simulink model "Rebuild"  (R2024b)
settings: Solver=VariableStepAuto  StartTime=0.0  StopTime=12  RelTol=1e-3
values from neighbouring files (symbols this model uses):
  A = 1.1    [RT14e_Parameters.m]    (also in RT15e_Parameters.m = 1.088; RT15evo_Parameters.m = 1.088)
  Aero_balance = 55    [RT14e_Parameters.m]    (also in RT15e_Parameters.m; RT15evo_Parameters.m)
  Aeromaps_ON = 0    [SIM_setup.m]
  air_density = 1.2    [SIM_setup.m]
  Balance_FW = Data_FW_STD(1:end,2)    [RT15e_Parameters.m]    (also in RT15evo_Parameters.m)
  Balance_R_11 = Data_R_11(1:end,2)    [RT15e_Parameters.m]    (also in RT15evo_Parameters.m)
  Br_coef_of_friction_F = 0.33    [RT14e_Parameters.m]    (also in RT15e_Parameters.m; RT15evo_Parameters.m)
  Br_coef_of_friction_R = 0.33    [RT14e_Parameters.m]    (also in RT15e_Parameters.m; RT15evo_Parameters.m)
  Br_pistons_area_F = 3617.26/1e6    (= 0.00361726)    [RT14e_Parameters.m]    (also in RT15e_Parameters.m; RT15evo_Parameters.m)
  Br_pistons_area_R = 2026.83/1e6    (= 0.00202683)    [RT14e_Parameters.m]    (also in RT15e_Parameters.m; RT15evo_Parameters.m)
  CdA = 1.31*A    (= 1.441)    [RT14e_Parameters.m]    (also in RT15e_Parameters.m = 1.700544; RT15evo_Parameters.m = 1.700544)
  CdA_FW = Data_FW_STD(1:end,3)    [RT15e_Parameters.m]    (also in RT15evo_Parameters.m)
  CdA_R_11 = Data_R_11(1:end,3)    [RT15e_Parameters.m]    (also in RT15evo_Parameters.m)
  ClA = 3.3*A    (= 3.63)    [RT14e_Parameters.m]    (also in RT15e_Parameters.m = 4.36288; RT15evo_Parameters.m = 4.36288)
  ClA_FW = Data_FW_STD(1:end,4)    [RT15e_Parameters.m]    (also in RT15evo_Parameters.m)
  ClA_R_11 = Data_R_11(1:end,4)    [RT15e_Parameters.m]    (also in RT15evo_Parameters.m)
  CoG_z = 0.35    [RT14e_Parameters.m]    (also in RT15e_Parameters.m = 0.28495; RT15evo_Parameters.m = 0.28495)
  Default_Fz_FL = Default_Fz_F/2 + (Default_Fz_F*CoG_y/Track_Front)    [RT14e_Parameters.m]    (also in RT15e_Parameters.m; RT15evo_Parameters.m)
  Default_Fz_FR = Default_Fz_F/2 - (Default_Fz_F*CoG_y/Track_Front)    [RT14e_Parameters.m]    (also in RT15e_Parameters.m; RT15evo_Parameters.m)
  Default_Fz_RL = Default_Fz_R/2 + (Default_Fz_R*CoG_y/Track_Rear)    [RT14e_Parameters.m]    (also in RT15e_Parameters.m; RT15evo_Parameters.m)
  Default_Fz_RR = Default_Fz_R/2 - (Default_Fz_R*CoG_y/Track_Rear)    [RT14e_Parameters.m]    (also in RT15e_Parameters.m; RT15evo_Parameters.m)
  Effective_br_disk_r_F = 0.0905    [RT14e_Parameters.m]    (also in RT15e_Parameters.m; RT15evo_Parameters.m)
  Effective_br_disk_r_R = 0.0895    [RT14e_Parameters.m]    (also in RT15e_Parameters.m; RT15evo_Parameters.m)
  Front_brake_balance = 0.0    (= 0)    [RT14e_Parameters.m]    (also in RT15e_Parameters.m; RT15evo_Parameters.m)
  Front_brake_pump_area = 153.94    [RT14e_Parameters.m]    (also in RT15e_Parameters.m; RT15evo_Parameters.m)
  Front_desired_brake_p_balance = 0.6    [RT14e_Parameters.m]    (also in RT15e_Parameters.m; RT15evo_Parameters.m)
  FW_Setup = Data_FW_STD(1:end,1)    [RT15e_Parameters.m]    (also in RT15evo_Parameters.m)
  Fx = Data_Fx(2:end,3:end)    [RT14e_Parameters.m]    (also in RT15e_Parameters.m; RT15evo_Parameters.m)
  Fy = Data_Fy(2:end,3:end)    [RT14e_Parameters.m]    (also in RT15e_Parameters.m; RT15evo_Parameters.m)
  Fz = Data_Fy(2:end,2)    [RT14e_Parameters.m]    (also in RT15e_Parameters.m; RT15evo_Parameters.m)
  g = 9.81    [SIM_setup.m]
  Gear_ratio = 12.9    [RT14e_Parameters.m]    (also in RT15e_Parameters.m; RT15evo_Parameters.m)
  Iz_wehicle = 120    [RT14e_Parameters.m]    (also in RT15e_Parameters.m; RT15evo_Parameters.m)
  Iz_wheel = 0.15    [RT14e_Parameters.m]    (also in RT15e_Parameters.m; RT15evo_Parameters.m)
  Lf = Wheelbase - CoG_x    (= 0.77)    [RT14e_Parameters.m]    (also in RT15e_Parameters.m = 0.7504; RT15evo_Parameters.m = 0.7504)
  LLTD = 0.45    [RT14e_Parameters.m]    (also in RT15e_Parameters.m = 0.55; RT15evo_Parameters.m = 0.55)
  Lock_brake_balance = false    [RT14e_Parameters.m]    (also in RT15e_Parameters.m; RT15evo_Parameters.m)
  Lr = Wheelbase - Lf    (= 0.755)    [RT14e_Parameters.m]    (also in RT15e_Parameters.m = 0.7746; RT15evo_Parameters.m = 0.7746)
  Mass = Vehicle_mass + Driver_mass    (= 290)    [RT14e_Parameters.m]    (also in RT15e_Parameters.m = 265; RT15evo_Parameters.m)
  Motor_maximum_power = 35366    [RT14e_Parameters.m]    (also in RT15e_Parameters.m; RT15evo_Parameters.m)
  RB_torque_setting_1 = -2    [RT14e_Parameters.m]    (also in RT15e_Parameters.m; RT15evo_Parameters.m)
  RB_torque_setting_10 = -20    [RT14e_Parameters.m]    (also in RT15e_Parameters.m; RT15evo_Parameters.m)
  RB_torque_setting_2 = -4    [RT14e_Parameters.m]    (also in RT15e_Parameters.m; RT15evo_Parameters.m)
  RB_torque_setting_3 = -6    [RT14e_Parameters.m]    (also in RT15e_Parameters.m; RT15evo_Parameters.m)
  RB_torque_setting_4 = -8    [RT14e_Parameters.m]    (also in RT15e_Parameters.m; RT15evo_Parameters.m)
  RB_torque_setting_5 = -10    [RT14e_Parameters.m]    (also in RT15e_Parameters.m; RT15evo_Parameters.m)
  RB_torque_setting_6 = -12    [RT14e_Parameters.m]    (also in RT15e_Parameters.m; RT15evo_Parameters.m)
  RB_torque_setting_7 = -14    [RT14e_Parameters.m]    (also in RT15e_Parameters.m; RT15evo_Parameters.m)
  RB_torque_setting_8 = -16    [RT14e_Parameters.m]    (also in RT15e_Parameters.m; RT15evo_Parameters.m)
  RB_torque_setting_9 = -18    [RT14e_Parameters.m]    (also in RT15e_Parameters.m; RT15evo_Parameters.m)
  Rear_brake_pump_area = 198.56    [RT14e_Parameters.m]    (also in RT15e_Parameters.m; RT15evo_Parameters.m)
  Roll_Angle_11 = Data_R_11(1:end,1)    [RT15e_Parameters.m]    (also in RT15evo_Parameters.m)
  SA = Data_Fy(1,3:end)    [RT14e_Parameters.m]    (also in RT15e_Parameters.m; RT15evo_Parameters.m)
  SR = Data_Fx(1,3:end)    [RT14e_Parameters.m]    (also in RT15e_Parameters.m; RT15evo_Parameters.m)
  start_acc_x = double(start_acc_x_ts.Data)    [SIM_setup.m]
  start_acc_y = double(start_acc_y_ts.Data)    [SIM_setup.m]
  start_time = 1188    [SIM_setup.m]
  start_velocity_x = double(start_velocity_x_ts.Data)    [SIM_setup.m]
  start_velocity_y = double(start_velocity_y_ts.Data)    [SIM_setup.m]
  start_yaw_acc = double(start_yaw_acc_ts.Data)    [SIM_setup.m]
  start_yaw_rate = double(start_yaw_rate_ts.Data)    [SIM_setup.m]
  Static_Camber_FL = 0    [RT14e_Parameters.m]    (also in RT15e_Parameters.m; RT15evo_Parameters.m)
  Static_Camber_FR = 0    [RT14e_Parameters.m]    (also in RT15e_Parameters.m; RT15evo_Parameters.m)
  Static_Camber_RL = 0    [RT14e_Parameters.m]    (also in RT15e_Parameters.m; RT15evo_Parameters.m)
  Static_Camber_RR = 0    [RT14e_Parameters.m]    (also in RT15e_Parameters.m; RT15evo_Parameters.m)
  Static_Toe_FL = 0    [RT14e_Parameters.m]    (also in RT15e_Parameters.m; RT15evo_Parameters.m)
  Static_Toe_FR = 0    [RT14e_Parameters.m]    (also in RT15e_Parameters.m; RT15evo_Parameters.m)
  Static_Toe_RL = 0    [RT14e_Parameters.m]    (also in RT15e_Parameters.m; RT15evo_Parameters.m)
  Static_Toe_RR = 0    [RT14e_Parameters.m]    (also in RT15e_Parameters.m; RT15evo_Parameters.m)
  Steering_Angle_FL = Data_Steering(1:end,2)    [RT14e_Parameters.m]    (also in RT15e_Parameters.m; RT15evo_Parameters.m)
  Steering_Angle_FR = Data_Steering(1:end,3)    [RT14e_Parameters.m]    (also in RT15e_Parameters.m; RT15evo_Parameters.m)
  Steering_Wheel_Angle = Data_Steering(1:end,1)    [RT14e_Parameters.m]    (also in RT15e_Parameters.m; RT15evo_Parameters.m)
  Tire_radius = 0.203    [RT14e_Parameters.m]    (also in RT15e_Parameters.m; RT15evo_Parameters.m)
  Torque_limit_2 = Motor_maximum_torque*0.2    (= 5.82)    [RT14e_Parameters.m]    (also in RT15e_Parameters.m; RT15evo_Parameters.m)
  Torque_limit_3 = Motor_maximum_torque*0.3    (= 8.73)    [RT14e_Parameters.m]    (also in RT15e_Parameters.m; RT15evo_Parameters.m)
  Torque_limit_4 = Motor_maximum_torque*0.4    (= 11.64)    [RT14e_Parameters.m]    (also in RT15e_Parameters.m; RT15evo_Parameters.m)
  Torque_limit_5 = Motor_maximum_torque*0.5    (= 14.55)    [RT14e_Parameters.m]    (also in RT15e_Parameters.m; RT15evo_Parameters.m)
  Torque_limit_6 = Motor_maximum_torque*0.6    (= 17.46)    [RT14e_Parameters.m]    (also in RT15e_Parameters.m; RT15evo_Parameters.m)
  Torque_limit_7 = Motor_maximum_torque*0.7    (= 20.37)    [RT14e_Parameters.m]    (also in RT15e_Parameters.m; RT15evo_Parameters.m)
  Torque_limit_8 = Motor_maximum_torque*0.8    (= 23.28)    [RT14e_Parameters.m]    (also in RT15e_Parameters.m; RT15evo_Parameters.m)
  Torque_limit_9 = 29.1    [RT14e_Parameters.m]    (also in RT15e_Parameters.m; RT15evo_Parameters.m)
  Torque_limit_max = Motor_maximum_torque    (= 29.1)    [RT14e_Parameters.m]    (also in RT15e_Parameters.m; RT15evo_Parameters.m)
  Torque_limit_min = Motor_maximum_torque*0.1    (= 2.91)    [RT14e_Parameters.m]    (also in RT15e_Parameters.m; RT15evo_Parameters.m)
  Torque_limit_set = 10    [RT14e_Parameters.m]    (also in RT15e_Parameters.m; RT15evo_Parameters.m)
  Track_Front = 1.2    [RT14e_Parameters.m]    (also in RT15e_Parameters.m; RT15evo_Parameters.m)
  Track_Rear = 1.18    [RT14e_Parameters.m]    (also in RT15e_Parameters.m; RT15evo_Parameters.m)
  TV_ON = 0    [SIM_setup.m]
  TV_RB_understeer_gradient_1 = -0.5    [RT14e_Parameters.m]    (also in RT15e_Parameters.m; RT15evo_Parameters.m)
  TV_RB_understeer_gradient_10 = 0.005    [RT14e_Parameters.m]    (also in RT15e_Parameters.m; RT15evo_Parameters.m)
  TV_RB_understeer_gradient_2 = -0.1    [RT14e_Parameters.m]    (also in RT15e_Parameters.m; RT15evo_Parameters.m)
  TV_RB_understeer_gradient_3 = 0.08    [RT14e_Parameters.m]    (also in RT15e_Parameters.m; RT15evo_Parameters.m)
  TV_RB_understeer_gradient_4 = 0.06    [RT14e_Parameters.m]    (also in RT15e_Parameters.m; RT15evo_Parameters.m)
  TV_RB_understeer_gradient_5 = 0.05    [RT14e_Parameters.m]    (also in RT15e_Parameters.m; RT15evo_Parameters.m)
  TV_RB_understeer_gradient_6 = 0.04    [RT14e_Parameters.m]    (also in RT15e_Parameters.m; RT15evo_Parameters.m)
  TV_RB_understeer_gradient_7 = 0.03    [RT14e_Parameters.m]    (also in RT15e_Parameters.m; RT15evo_Parameters.m)
  TV_RB_understeer_gradient_8 = 0.02    [RT14e_Parameters.m]    (also in RT15e_Parameters.m; RT15evo_Parameters.m)
  TV_RB_understeer_gradient_9 = 0.01    [RT14e_Parameters.m]    (also in RT15e_Parameters.m; RT15evo_Parameters.m)
  TV_understeer_gradient_1 = -0.5    [RT14e_Parameters.m]    (also in RT15e_Parameters.m; RT15evo_Parameters.m)
  TV_understeer_gradient_10 = 0.002    [RT14e_Parameters.m]    (also in RT15e_Parameters.m; RT15evo_Parameters.m)
  TV_understeer_gradient_2 = -0.1    [RT14e_Parameters.m]    (also in RT15e_Parameters.m; RT15evo_Parameters.m)
  TV_understeer_gradient_3 = 0.06    [RT14e_Parameters.m]    (also in RT15e_Parameters.m; RT15evo_Parameters.m)
  TV_understeer_gradient_4 = 0.05    [RT14e_Parameters.m]    (also in RT15e_Parameters.m; RT15evo_Parameters.m)
  TV_understeer_gradient_5 = 0.04    [RT14e_Parameters.m]    (also in RT15e_Parameters.m; RT15evo_Parameters.m)
  TV_understeer_gradient_6 = 0.03    [RT14e_Parameters.m]    (also in RT15e_Parameters.m; RT15evo_Parameters.m)
  TV_understeer_gradient_7 = 0.02    [RT14e_Parameters.m]    (also in RT15e_Parameters.m; RT15evo_Parameters.m)
  TV_understeer_gradient_8 = 0.01    [RT14e_Parameters.m]    (also in RT15e_Parameters.m; RT15evo_Parameters.m)
  TV_understeer_gradient_9 = 0.005    [RT14e_Parameters.m]    (also in RT15e_Parameters.m; RT15evo_Parameters.m)
  Vx_APPS_ON = 1    [SIM_setup.m]
  Wheel_rolling_resistance = 0.055    [RT14e_Parameters.m]    (also in RT15e_Parameters.m; RT15evo_Parameters.m)
  Wheelbase = 1.525    [RT14e_Parameters.m]    (also in RT15e_Parameters.m; RT15evo_Parameters.m)
undefined symbols (not defined in the file or in its folder): Actual_Torque_Value_RL, Actual_Torque_Value_RR, aero_balance, APPS, Brake_Pressure_Front, Brake_Pressure_Rear, Cl, lateral_load_transfer_distribution, maths_GPS_Velocity, Max_Torque, rad, s, Steering_position, tire_radius, wheel_base, Wheel_Speed_RL, Wheel_Speed_RR, Xsens_MTI_670_accX, Xsens_MTI_670_accY, Xsens_MTI_670_gyrZ
libraries: simulink x30, simulink_extras x11, slpidlib x9, dspstat3 x4, slrealtimeloglib x1, aerolibconvert2 x1
(part 3 of 6)

== system Rebuild/Main/Wheels & Tires/Wheel Speeds/Wheel Speed RL ==
  Rolling Resistance : Inport
  Fx [N] : Inport  Port=2
  Torque [Nm] : Inport  Port=3
  Add1 : Sum  Inputs=--+-
  Bus Selector : BusSelector  OutputSignals=Brake Torque [Nm].Brake Torque RL [Nm],Motor Torque [Nm].Motor Torque RL [Nm]
  Bus Selector1 : BusSelector  OutputSignals=Rolling Resistance RL
  Bus Selector2 : BusSelector  OutputSignals=Fx RL [N]
  Constant4 : Constant  Value=Tire_radius
  Gain : Gain  Gain=Gear_ratio
  Gain1 : Gain  Gain=1/Iz_wheel
  Integrator2 : Integrator  InitialCondition=start_velocity_x / Tire_radius
  Product : Product
  Saturation : Saturate  UpperLimit=200  LowerLimit=-20
  Wheel Speed RL [rad/s] : Outport
  wires:
  Fx [N]/1 -> Bus Selector2/1
  Bus Selector2/1 -> Product/2  "<Fx RL [N]>"
  Rolling Resistance/1 -> Bus Selector1/1
  Saturation/1 -> Wheel Speed RL [rad/s]/1
  Torque [Nm]/1 -> Bus Selector/1
  Bus Selector1/1 -> Add1/4  "<Rolling Resistance RL>"
  Bus Selector/1 -> Add1/2  "<Brake Torque RL [Nm]>"
  Gain1/1 -> Integrator2/1
  Integrator2/1 -> Saturation/1
  Product/1 -> Add1/1
  Add1/1 -> Gain1/1
  Constant4/1 -> Product/1
  Bus Selector/2 -> Gain/1  "<Motor Torque RL [Nm]>"
  Gain/1 -> Add1/3

== system Rebuild/Main/Wheels & Tires/Wheel Speeds/Wheel Speed RR ==
  Rolling Resistance : Inport
  Fx [N] : Inport  Port=2
  Torque [Nm] : Inport  Port=3
  Add1 : Sum  Inputs=--+-
  Bus Selector : BusSelector  OutputSignals=Brake Torque [Nm].Brake Torque RR [Nm],Motor Torque [Nm].Motor Torque RR [Nm]
  Bus Selector1 : BusSelector  OutputSignals=Rolling Resistance RR
  Bus Selector2 : BusSelector  OutputSignals=Fx RR [N]
  Constant4 : Constant  Value=Tire_radius
  Gain : Gain  Gain=Gear_ratio
  Gain1 : Gain  Gain=1/Iz_wheel
  Integrator2 : Integrator  InitialCondition=start_velocity_x / Tire_radius
  Product : Product
  Saturation : Saturate  UpperLimit=200  LowerLimit=-20
  Wheel Speed RL [rad/s] : Outport
  wires:
  Bus Selector/2 -> Gain/1  "<Motor Torque RR [Nm]>"
  Add1/1 -> Gain1/1
  Integrator2/1 -> Saturation/1
  Gain1/1 -> Integrator2/1
  Bus Selector2/1 -> Product/2  "<Fx RR [N]>"
  Fx [N]/1 -> Bus Selector2/1
  Bus Selector/1 -> Add1/2  "<Brake Torque RR [Nm]>"
  Bus Selector1/1 -> Add1/4  "<Rolling Resistance RR>"
  Constant4/1 -> Product/1
  Product/1 -> Add1/1
  Torque [Nm]/1 -> Bus Selector/1
  Rolling Resistance/1 -> Bus Selector1/1
  Saturation/1 -> Wheel Speed RL [rad/s]/1
  Gain/1 -> Add1/3

== system Rebuild/Main/Powertrain/Motors/Control Algorithms/ABS ==
  Brake_Torque [Nm] : Inport
  Slip_Ratio : Inport  Port=2
  ABS_FL : Subsystem
  ABS_FR : Subsystem
  ABS_RL : Subsystem
  ABS_RR : Subsystem
  Bus Creator : BusCreator  Inputs=4
  Bus Selector : BusSelector  OutputSignals=Front.FL,Front.FR,Rear.RL,Rear.RR
  Bus Selector1 : BusSelector  OutputSignals=Slip_Ratio_FL,Slip_Ratio_FR,Slip_Ratio_RL,Slip_Ratio_RR
  ABS_Torque : Outport
  wires:
  Brake_Torque [Nm]/1 -> Bus Selector/1
  Slip_Ratio/1 -> Bus Selector1/1
  Bus Selector/1 -> ABS_FL/1(Torque IN)  "<FL>"
  Bus Selector1/1 -> ABS_FL/2(Slip_Ratio)  "<Slip_Ratio_FL>"
  Bus Selector/2 -> ABS_FR/1(Torque IN)  "<FR>"
  Bus Selector1/2 -> ABS_FR/2(Slip_Ratio)  "<Slip_Ratio_FR>"
  Bus Selector/3 -> ABS_RL/1(Torque IN)  "<RL>"
  Bus Selector1/3 -> ABS_RL/2(Slip_Ratio)  "<Slip_Ratio_RL>"
  Bus Selector/4 -> ABS_RR/1(Torque IN)  "<RR>"
  Bus Selector1/4 -> ABS_RR/2(Slip_Ratio)  "<Slip_Ratio_RR>"
  ABS_FL/1(ABS Torque OUT) -> Bus Creator/1  "FL"
  ABS_FR/1(ABS Torque OUT) -> Bus Creator/2  "FR"
  ABS_RL/1(ABS Torque OUT) -> Bus Creator/3  "RL"
  ABS_RR/1(ABS Torque OUT) -> Bus Creator/4  "RR"
  Bus Creator/1 -> ABS_Torque/1  "ABS_Torque"

== system Rebuild/Main/Powertrain/Motors/Control Algorithms/ABS1 ==
  Brake_Torque [Nm] : Inport
  Slip_Ratio : Inport  Port=2
  ABS_FL1 : Subsystem
  ABS_FR1 : Subsystem
  ABS_RL1 : Subsystem
  ABS_RR1 : Subsystem
  Bus Creator2 : BusCreator  Inputs=4
  Bus Selector2 : BusSelector  OutputSignals=Front.FL,Front.FR,Rear.RL,Rear.RR
  Bus Selector3 : BusSelector  OutputSignals=Slip_Ratio_FL,Slip_Ratio_FR,Slip_Ratio_RL,Slip_Ratio_RR
  ABS_Torque : Outport
  wires:
  Bus Creator2/1 -> ABS_Torque/1  "ABS_Torque"
  Bus Selector3/3 -> ABS_RL1/2(Slip_Ratio)  "<Slip_Ratio_RL>"
  Bus Selector3/2 -> ABS_FR1/2(Slip_Ratio)  "<Slip_Ratio_FR>"
  ABS_RR1/1(ABS Torque OUT) -> Bus Creator2/4  "RR"
  Bus Selector2/3 -> ABS_RL1/1(Torque IN)  "<RL>"
  Bus Selector2/2 -> ABS_FR1/1(Torque IN)  "<FR>"
  Bus Selector2/4 -> ABS_RR1/1(Torque IN)  "<RR>"
  ABS_FL1/1(ABS Torque OUT) -> Bus Creator2/1  "FL"
  ABS_FR1/1(ABS Torque OUT) -> Bus Creator2/2  "FR"
  Bus Selector3/4 -> ABS_RR1/2(Slip_Ratio)  "<Slip_Ratio_RR>"
  ABS_RL1/1(ABS Torque OUT) -> Bus Creator2/3  "RL"
  Bus Selector3/1 -> ABS_FL1/2(Slip_Ratio)  "<Slip_Ratio_FL>"
  Bus Selector2/1 -> ABS_FL1/1(Torque IN)  "<FL>"
  Brake_Torque [Nm]/1 -> Bus Selector2/1
  Slip_Ratio/1 -> Bus Selector3/1

== system Rebuild/Main/Powertrain/Motors/Control Algorithms/TV Algorithm ==
  Brakes : Inport
  Positive Torque Command [Nm] : Inport  Port=2
  States : Inport  Port=3
  Wheel Angle F [deg] : Inport  Port=4
  Bus Selector : BusSelector  OutputSignals=Yaw_Rate [rad/s],Y,X,V_x [m/s],V_y [m/s]
  Radians to Degrees : simulink_extras/Transformations/Radians to Degrees
  Subsystem : Subsystem
  Torque Vectoring : Subsystem
  Commanded Torque RL [Nm] : Outport
  Commanded Torque RR [Nm] : Outport  Port=2
  wires:
  States/1 -> Bus Selector/1
  Bus Selector/1 -> Radians to Degrees/1  "<Yaw_Rate [rad/s]>"
  Torque Vectoring/1(Torque After TV RL [Nm]) -> Commanded Torque RL [Nm]/1  "Torque After TV RL [Nm]"
  Torque Vectoring/2(Torque After TV RR [Nm]) -> Commanded Torque RR [Nm]/1  "Torque After TV RL [Nm]"
  Wheel Angle F [deg]/1 -> Torque Vectoring/8(Wheel Angle F [deg])
  Bus Selector/2 -> Torque Vectoring/5(Xsens accY [m/s2])  "<Y>"
  Bus Selector/3 -> Torque Vectoring/6(Xsens accX [m/s2])  "<X>"
  Bus Selector/4 -> Torque Vectoring/9(Vehicle Speed [km/h])  "<V_x [m/s]>"
  Positive Torque Command [Nm]/1 -> Torque Vectoring/2(Positive Torque Command RR [Nm]), Torque Vectoring/1(Positive Torque Command RL [Nm])
  Brakes/1 -> Torque Vectoring/7(Brakes)

== system Rebuild/Main/Powertrain/Motors/Power Limit/Power Calculation ==
  In1 : Inport
  Bus Creator : BusCreator  Inputs=4
  Bus Selector : BusSelector  OutputSignals=Motor Torque FL after TV [Nm]
  Bus Selector1 : BusSelector  OutputSignals=Motor Torque FR after TV [Nm]
  Bus Selector2 : BusSelector  OutputSignals=Wheel Speeds.Wheel Speeds [rad/s].Wheel Speed FL [rad/s]
  Bus Selector3 : BusSelector  OutputSignals=Wheel Speeds.Wheel Speeds [rad/s].Wheel Speed FR [rad/s]
  Bus Selector4 : BusSelector  OutputSignals=Motor Torque RL after TV [Nm]
  Bus Selector5 : BusSelector  OutputSignals=Wheel Speeds.Wheel Speeds [rad/s].Wheel Speed RL [rad/s]
  Bus Selector6 : BusSelector  OutputSignals=Motor Torque RR after TV [Nm]
  Bus Selector7 : BusSelector  OutputSignals=Wheel Speeds.Wheel Speeds [rad/s].Wheel Speed RR [rad/s]
  Gain{,1..3} (4 alike) : Gain  Gain=Gear_ratio
  Product{,1..3} (4 alike) : Product
  Motor Power [W] : Outport
  wires:
  Bus Selector/1 -> Product/1  "<Motor Torque FL after TV [Nm]>"
  In1/1 -> Bus Selector6/1, Bus Selector4/1, Bus Selector1/1, Bus Selector/1
  Bus Selector7/1 -> Gain3/1  "<Wheel Speed RR [rad/s]>"
  [Tires] -> Bus Selector7/1, Bus Selector5/1, Bus Selector3/1, Bus Selector2/1
  Product3/1 -> Bus Creator/4  "Motor Power RR [W]"
  Bus Selector2/1 -> Gain/1  "<Wheel Speed FL [rad/s]>"
  Gain/1 -> Product/2
  Bus Selector1/1 -> Product1/1  "<Motor Torque FR after TV [Nm]>"
  Bus Creator/1 -> Motor Power [W]/1  "Motor Power [W]"
  Gain3/1 -> Product3/2
  Bus Selector6/1 -> Product3/1  "<Motor Torque RR after TV [Nm]>"
  Product2/1 -> Bus Creator/3  "Motor Power RL [W]"
  Gain2/1 -> Product2/2
  Bus Selector5/1 -> Gain2/1  "<Wheel Speed RL [rad/s]>"
  Bus Selector4/1 -> Product2/1  "<Motor Torque RL after TV [Nm]>"
  Product1/1 -> Bus Creator/2  "Motor Power FR [W]"
  Product/1 -> Bus Creator/1  "Motor Power FL [W]"
  Gain1/1 -> Product1/2
  Bus Selector3/1 -> Gain1/1  "<Wheel Speed FR [rad/s]>"

== system Rebuild/Main/Powertrain/Motors/Regen Braking/Subsystem ==
  Brake_Preasure_Front : Inport
  Brake_Preasure_Rear : Inport  Port=2
  Desired_Brake_Balance : Inport  Port=3
  Divide2 : Product  Inputs=*/
  Front_Pump_Area : Constant  Value=Front_brake_pump_area
  Product2 : Product
  Product3 : Product
  Product4 : Product
  Rear_Pump_Area : Constant  Value=Rear_brake_pump_area
  Subtract2 : Sum  Inputs=+-
  Sum1 : Sum  Inputs=+-|
  "Motor_Rear_\"Preasure\"" : Outport
  wires:
  Product4/1 -> Sum1/1, Product2/1
  Brake_Preasure_Front/1 -> Product4/1
  Rear_Pump_Area/1 -> Product3/2
  Product3/1 -> Divide2/2
  Product2/1 -> Sum1/2
  Divide2/1 -> Subtract2/1
  Sum1/1 -> Divide2/1
  Front_Pump_Area/1 -> Product4/2
  Desired_Brake_Balance/1 -> Product3/1, Product2/2
  Subtract2/1 -> "Motor_Rear_\"Preasure\""/1
  Brake_Preasure_Rear/1 -> Subtract2/2

== system Rebuild/Main/Powertrain/Motors/Torque Command [Nm]/Switch Case Action Subsystem ==
  APPS : Inport
  Action Port : ActionPort  ActionPortLabel=default:
  1-D Lookup Table1 : Lookup_n-D  NumberOfTableDimensions=1  BreakpointsForDimension1=[0 100]  Table=[0 Torque_limit_max]  InternalRulePriority=Speed  RndMeth=Simplest
  Out1 : Outport
  wires:
  APPS/1 -> 1-D Lookup Table1/1
  1-D Lookup Table1/1 -> Out1/1

== system Rebuild/Main/Powertrain/Motors/Torque Command [Nm]/Switch Case Action Subsystem1 ==
  APPS : Inport
  Action Port : ActionPort  ActionPortLabel=case [ 10 ]:
  1-D Lookup Table1 : Lookup_n-D  NumberOfTableDimensions=1  BreakpointsForDimension1=[0 100]  Table=[0 Torque_limit_max]  InternalRulePriority=Speed  RndMeth=Simplest
  Out1 : Outport
  wires:
  1-D Lookup Table1/1 -> Out1/1
  APPS/1 -> 1-D Lookup Table1/1

== system Rebuild/Main/Powertrain/Motors/Torque Command [Nm]/Switch Case Action Subsystem10 ==
  APPS : Inport
  Action Port : ActionPort  ActionPortLabel=case [ 1 ]:
  1-D Lookup Table1 : Lookup_n-D  NumberOfTableDimensions=1  BreakpointsForDimension1=[0 100]  Table=[0 Torque_limit_min]  InternalRulePriority=Speed  RndMeth=Simplest
  Out1 : Outport
  wires:
  1-D Lookup Table1/1 -> Out1/1
  APPS/1 -> 1-D Lookup Table1/1

== system Rebuild/Main/Powertrain/Motors/Torque Command [Nm]/Switch Case Action Subsystem2 ==
  APPS : Inport
  Action Port : ActionPort  ActionPortLabel=case [ 9 ]:
  1-D Lookup Table1 : Lookup_n-D  NumberOfTableDimensions=1  BreakpointsForDimension1=[0 100]  Table=[0 Torque_limit_9]  InternalRulePriority=Speed  RndMeth=Simplest
  Out1 : Outport
  wires:
  APPS/1 -> 1-D Lookup Table1/1
  1-D Lookup Table1/1 -> Out1/1

== system Rebuild/Main/Powertrain/Motors/Torque Command [Nm]/Switch Case Action Subsystem3 ==
  APPS : Inport
  Action Port : ActionPort  ActionPortLabel=case [ 8 ]:
  1-D Lookup Table1 : Lookup_n-D  NumberOfTableDimensions=1  BreakpointsForDimension1=[0 100]  Table=[0 Torque_limit_8]  InternalRulePriority=Speed  RndMeth=Simplest
  Out1 : Outport
  wires:
  1-D Lookup Table1/1 -> Out1/1
  APPS/1 -> 1-D Lookup Table1/1

== system Rebuild/Main/Powertrain/Motors/Torque Command [Nm]/Switch Case Action Subsystem4 ==
  APPS : Inport
  Action Port : ActionPort  ActionPortLabel=case [ 7 ]:
  1-D Lookup Table1 : Lookup_n-D  NumberOfTableDimensions=1  BreakpointsForDimension1=[0 100]  Table=[0 Torque_limit_7]  InternalRulePriority=Speed  RndMeth=Simplest
  Out1 : Outport
  wires:
  APPS/1 -> 1-D Lookup Table1/1
  1-D Lookup Table1/1 -> Out1/1

== system Rebuild/Main/Powertrain/Motors/Torque Command [Nm]/Switch Case Action Subsystem5 ==
  APPS : Inport
  Action Port : ActionPort  ActionPortLabel=case [ 6 ]:
  1-D Lookup Table1 : Lookup_n-D  NumberOfTableDimensions=1  BreakpointsForDimension1=[0 100]  Table=[0 Torque_limit_6]  InternalRulePriority=Speed  RndMeth=Simplest
  Out1 : Outport
  wires:
  1-D Lookup Table1/1 -> Out1/1
  APPS/1 -> 1-D Lookup Table1/1

== system Rebuild/Main/Powertrain/Motors/Torque Command [Nm]/Switch Case Action Subsystem6 ==
  APPS : Inport
  Action Port : ActionPort  ActionPortLabel=case [ 5 ]:
  1-D Lookup Table1 : Lookup_n-D  NumberOfTableDimensions=1  BreakpointsForDimension1=[0 100]  Table=[0 Torque_limit_5]  InternalRulePriority=Speed  RndMeth=Simplest
  Out1 : Outport
  wires:
  1-D Lookup Table1/1 -> Out1/1
  APPS/1 -> 1-D Lookup Table1/1

== system Rebuild/Main/Powertrain/Motors/Torque Command [Nm]/Switch Case Action Subsystem7 ==
  APPS : Inport
  Action Port : ActionPort  ActionPortLabel=case [ 4 ]:
  1-D Lookup Table1 : Lookup_n-D  NumberOfTableDimensions=1  BreakpointsForDimension1=[0 100]  Table=[0 Torque_limit_4]  InternalRulePriority=Speed  RndMeth=Simplest
  Out1 : Outport
  wires:
  APPS/1 -> 1-D Lookup Table1/1
  1-D Lookup Table1/1 -> Out1/1

== system Rebuild/Main/Powertrain/Motors/Torque Command [Nm]/Switch Case Action Subsystem8 ==
  APPS : Inport
  Action Port : ActionPort  ActionPortLabel=case [ 3 ]:
  1-D Lookup Table1 : Lookup_n-D  NumberOfTableDimensions=1  BreakpointsForDimension1=[0 100]  Table=[0 Torque_limit_3]  InternalRulePriority=Speed  RndMeth=Simplest
  Out1 : Outport
  wires:
  1-D Lookup Table1/1 -> Out1/1
  APPS/1 -> 1-D Lookup Table1/1

== system Rebuild/Main/Powertrain/Motors/Torque Command [Nm]/Switch Case Action Subsystem9 ==
  APPS : Inport
  Action Port : ActionPort  ActionPortLabel=case [ 2 ]:
  1-D Lookup Table1 : Lookup_n-D  NumberOfTableDimensions=1  BreakpointsForDimension1=[0 100]  Table=[0 Torque_limit_2]  InternalRulePriority=Speed  RndMeth=Simplest
  Out1 : Outport
  wires:
  APPS/1 -> 1-D Lookup Table1/1
  1-D Lookup Table1/1 -> Out1/1

== system Rebuild/Main/Wheels & Tires/Brakes/Brake_Balance_Adjustment/Enabled Subsystem ==
  In1 : Inport
  Enable : EnablePort
  Out1 : Outport  InitialOutput=[0.5]
  wires:
  In1/1 -> Out1/1

== system Rebuild/Main/Wheels & Tires/Slip Ratio & Slip Angle Calculation/Slip Angle/Slip Angle FL ==
  X Velocity [m/s] : Inport
  Y Velocity [m/s] : Inport  Port=2
  Yaw Rate [rad/s] : Inport  Port=3
  Steering Angle FL [rad] : Inport  Port=4
  Atan : Trigonometry  Operator=atan
  Constant : Constant  Value=Lf
  Constant1 : Constant  Value=Track_Front
  Divide : Product  Inputs=*/
  Gain : Gain  Gain=1/2
  Product : Product
  Product1 : Product
  Subtract : Sum
  Subtract1 : Sum
  Subtract2 : Sum  Inputs=+-
  Slip Angle FL [rad] : Outport
  wires:
  Subtract/1 -> Divide/1
  Product/1 -> Subtract/2
  Steering Angle FL [rad]/1 -> Subtract2/2
  Subtract1/1 -> Divide/2
  Constant1/1 -> Gain/1
  Yaw Rate [rad/s]/1 -> Product/2, Product1/1
  Gain/1 -> Product1/2
  Divide/1 -> Atan/1
  X Velocity [m/s]/1 -> Subtract1/2
  Y Velocity [m/s]/1 -> Subtract/1
  Product1/1 -> Subtract1/1
  Subtract2/1 -> Slip Angle FL [rad]/1
  Constant/1 -> Product/1
  Atan/1 -> Subtract2/1

== system Rebuild/Main/Wheels & Tires/Slip Ratio & Slip Angle Calculation/Slip Angle/Slip Angle FR ==
  X Velocity [m/s] : Inport
  Y Velocity [m/s] : Inport  Port=2
  Yaw Rate [rad/s] : Inport  Port=3
  Steering Angle FR [rad] : Inport  Port=4
  Atan : Trigonometry  Operator=atan
  Constant : Constant  Value=Lf
  Constant1 : Constant  Value=Track_Front
  Divide : Product  Inputs=*/
  Gain : Gain  Gain=1/2
  Product : Product
  Product1 : Product
  Subtract : Sum
  Subtract1 : Sum  Inputs=-+
  Subtract2 : Sum  Inputs=+-
  Slip Angle FR [rad] : Outport
  wires:
  Subtract2/1 -> Slip Angle FR [rad]/1
  Product1/1 -> Subtract1/1
  Yaw Rate [rad/s]/1 -> Product/2, Product1/1
  Divide/1 -> Atan/1
  Y Velocity [m/s]/1 -> Subtract/1
  Gain/1 -> Product1/2
  X Velocity [m/s]/1 -> Subtract1/2
  Constant/1 -> Product/1
  Steering Angle FR [rad]/1 -> Subtract2/2
  Product/1 -> Subtract/2
  Constant1/1 -> Gain/1
  Subtract1/1 -> Divide/2
  Subtract/1 -> Divide/1
  Atan/1 -> Subtract2/1

== system Rebuild/Main/Wheels & Tires/Slip Ratio & Slip Angle Calculation/Slip Angle/Slip Angle RL ==
  X Velocity [m/s] : Inport
  Y Velocity [m/s] : Inport  Port=2
  Yaw Rate [rad/s] : Inport  Port=3
  Steering Angle RL [rad] : Inport  Port=4
  Atan : Trigonometry  Operator=atan
  Constant : Constant  Value=Lr
  Constant1 : Constant  Value=Track_Rear
  Divide : Product  Inputs=*/
  Gain : Gain  Gain=1/2
  Product : Product
  Product1 : Product
  Subtract : Sum  Inputs=+-
  Subtract1 : Sum
  Subtract2 : Sum  Inputs=+-
  Slip Angle RL [rad] : Outport
  wires:
  X Velocity [m/s]/1 -> Subtract1/2
  Divide/1 -> Atan/1
  Product1/1 -> Subtract1/1
  Constant/1 -> Product/1
  Subtract2/1 -> Slip Angle RL [rad]/1
  Yaw Rate [rad/s]/1 -> Product/2, Product1/1
  Y Velocity [m/s]/1 -> Subtract/1
  Subtract/1 -> Divide/1
  Subtract1/1 -> Divide/2
  Product/1 -> Subtract/2
  Constant1/1 -> Gain/1
  Steering Angle RL [rad]/1 -> Subtract2/2
  Gain/1 -> Product1/2
  Atan/1 -> Subtract2/1

== system Rebuild/Main/Wheels & Tires/Slip Ratio & Slip Angle Calculation/Slip Angle/Slip Angle RR ==
  X Velocity [m/s] : Inport
  Y Velocity [m/s] : Inport  Port=2
  Yaw Rate [rad/s] : Inport  Port=3
  Steering Angle RR [rad] : Inport  Port=4
  Atan : Trigonometry  Operator=atan
  Constant : Constant  Value=Lr
  Constant1 : Constant  Value=Track_Rear
  Divide : Product  Inputs=*/
  Gain : Gain  Gain=1/2
  Product : Product
  Product1 : Product
  Subtract : Sum  Inputs=+-
  Subtract1 : Sum  Inputs=-+
  Subtract2 : Sum  Inputs=+-
  Slip Angle RR [rad] : Outport
  wires:
  Subtract/1 -> Divide/1
  Product/1 -> Subtract/2
  Steering Angle RR [rad]/1 -> Subtract2/2
  Subtract1/1 -> Divide/2
  Constant1/1 -> Gain/1
  Yaw Rate [rad/s]/1 -> Product/2, Product1/1
  Gain/1 -> Product1/2
  Divide/1 -> Atan/1
  X Velocity [m/s]/1 -> Subtract1/2
  Y Velocity [m/s]/1 -> Subtract/1
  Product1/1 -> Subtract1/1
  Subtract2/1 -> Slip Angle RR [rad]/1
  Constant/1 -> Product/1
  Atan/1 -> Subtract2/1

== system Rebuild/Main/Wheels & Tires/Slip Ratio & Slip Angle Calculation/Slip Ratio /Slip ratio FL ==
  Wheel Speed FL [rad/s] : Inport
  X Velocity [m/s] : Inport  Port=2
  Constant : Constant
  Constant4 : Constant  Value=Tire_radius
  Divide : Product  Inputs=**/
  Saturation : Saturate  UpperLimit=0.2
  Subtract : Sum  Inputs=+-
  Slip Ratio FL : Outport
  wires:
  Constant4/1 -> Divide/1
  X Velocity [m/s]/1 -> Divide/3
  Wheel Speed FL [rad/s]/1 -> Divide/2
  Constant/1 -> Subtract/2
  Subtract/1 -> Saturation/1
  Divide/1 -> Subtract/1
  Saturation/1 -> Slip Ratio FL/1

== system Rebuild/Main/Wheels & Tires/Slip Ratio & Slip Angle Calculation/Slip Ratio /Slip ratio FR ==
  Wheel Speed FR [rad/s] : Inport
  X Velocity [m/s] : Inport  Port=2
  Constant : Constant
  Constant4 : Constant  Value=Tire_radius
  Divide : Product  Inputs=**/
  Saturation : Saturate  UpperLimit=0.2
  Subtract : Sum  Inputs=+-
  Slip Ratio FR : Outport
  wires:
  Divide/1 -> Subtract/1
  Constant/1 -> Subtract/2
  Wheel Speed FR [rad/s]/1 -> Divide/2
  X Velocity [m/s]/1 -> Divide/3
  Subtract/1 -> Saturation/1
  Constant4/1 -> Divide/1
  Saturation/1 -> Slip Ratio FR/1

== system Rebuild/Main/Wheels & Tires/Slip Ratio & Slip Angle Calculation/Slip Ratio /Slip ratio RL ==
  Wheel Speed RL [rad/s] : Inport
  X Velocity [m/s] : Inport  Port=2
  Constant : Constant
  Constant4 : Constant  Value=Tire_radius
  Divide : Product  Inputs=**/
  Saturation : Saturate  UpperLimit=0.2
  Subtract : Sum  Inputs=+-
  Slip Ratio RL : Outport
  wires:
  Divide/1 -> Subtract/1
  Constant/1 -> Subtract/2
  Wheel Speed RL [rad/s]/1 -> Divide/2
  X Velocity [m/s]/1 -> Divide/3
  Constant4/1 -> Divide/1
  Subtract/1 -> Saturation/1
  Saturation/1 -> Slip Ratio RL/1

== system Rebuild/Main/Wheels & Tires/Slip Ratio & Slip Angle Calculation/Slip Ratio /Slip ratio RR ==
  Wheel Speed RR [rad/s] : Inport
  X Velocity [m/s] : Inport  Port=2
  Constant : Constant
  Constant4 : Constant  Value=Tire_radius
  Divide : Product  Inputs=**/
  Saturation : Saturate  UpperLimit=0.2
  Subtract : Sum  Inputs=+-
  Slip Ratio RR : Outport
  wires:
  Divide/1 -> Subtract/1
  Constant/1 -> Subtract/2
  Wheel Speed RR [rad/s]/1 -> Divide/2
  X Velocity [m/s]/1 -> Divide/3
  Constant4/1 -> Divide/1
  Subtract/1 -> Saturation/1
  Saturation/1 -> Slip Ratio RR/1

== system Rebuild/Main/Powertrain/Motors/Control Algorithms/ABS/ABS_FL ==
  Torque IN : Inport
  Slip_Ratio : Inport  Port=2
  Constant : Constant  Value=0.1
  Constant1 : Constant  Value=0.1
  Constant2 : Constant  Value=0.2
  Constant3 : Constant  Value=0
  Constant4 : Constant
  Gain : Gain  Gain=-1
  PID Controller : slpidlib/PID Controller  Controller=PI  Form=Ideal  TimeDomain=Continuous-time  UseExternalTs=off  SampleTime=-1  IntegratorMethod=Forward Euler  FilterMethod=Forward Euler  ControllerParametersSource=internal  P=100  I=10  UseKiTs=on  D=1  UseExternalDerivativeSource=off  N=100  UseFilter=on  TunerSelectOption=Transfer Function Based (PID Tuner App)  InitialConditionSource=internal  InitialConditionForIntegrator=0  InitialConditionForFilter=0  DifferentiatorICPrevScaledInput=0  ExternalReset=none  TrackingMode=off  Kt=1  LimitOutput=off  SatLimitsSource=internal  UpperSaturationLimit=inf  LowerSaturationLimit=-inf  LinearizeAsGain=on  AntiWindupMode=none  Kb=1  LimitIntegrator=off  UpperIntegratorSaturationLimit=inf  LowerIntegratorSaturationLimit=-inf  POutMin=[]  POutMax=[]  IOutMin=[]  IOutMax=[]  DOutMin=[]  DOutMax=[]  NOutMin=[]  NOutMax=[]  SumOutMin=[]  SumOutMax=[]  SaturationOutMin=[]  SaturationOutMax=[]  PParamMin=[]  PParamMax=[]  IParamMin=[]  IParamMax=[]  DParamMin=[]  DParamMax=[]  NParamMin=[]  NParamMax=[]  KbParamMin=[]  KbParamMax=[]  KtParamMin=[]  KtParamMax=[]  KbOutMin=[]  KbOutMax=[]  KtOutMin=[]  KtOutMax=[]  IntegratorOutMin=[]  IntegratorOutMax=[]  FilterOutMin=[]  FilterOutMax=[]  SumI1OutMin=[]  SumI1OutMax=[]  SumI2OutMin=[]  SumI2OutMax=[]  SumI3OutMin=[]  SumI3OutMax=[]  SumI4OutMin=[]  SumI4OutMax=[]  SumDOutMin=[]  SumDOutMax=[]  DifferentiatorOutMin=[]  DifferentiatorOutMax=[]  FilterDiffOutCoefMin=[]  FilterDiffOutCoefMax=[]  ReciprocalOutMin=[]  ReciprocalOutMax=[]  SumDenOutMin=[]  SumDenOutMax=[]  SumNumOutMin=[]  SumNumOutMax=[]  DivideOutMin=[]  DivideOutMax=[]  UdiffTsProdOutMin=[]  UdiffTsProdOutMax=[]  NTsProdOutMin=[]  NTsProdOutMax=[]  UintegralTsProdOutMin=[]  UintegralTsProdOutMax=[]  UngainTsProdOutMin=[]  UngainTsProdOutMax=[]  ClampingZeroOutDataTypeStr=Inherit: Inherit via back propagation  ClampingZeroOutMin=[]  ClampingZeroOutMax=[]  FilterDenConstantOutDataTypeStr=Inherit: Inherit via back propagation  FilterDenConstantOutMin=[]  FilterDenConstantOutMax=[]  PCopyOutDataTypeStr=Inherit: Inherit via back propagation  PCopyOutMin=[]  PCopyOutMax=[]  NCopyOutDataTypeStr=Inherit: Inherit via back propagation  NCopyOutMin=[]  NCopyOutMax=[]  IntegratorContinuousStateAttributes=''  IntegratorStateMustResolveToSignalObject=off  IntegratorRTWStateStorageClass=Auto  FilterContinuousStateAttributes=''  FilterStateMustResolveToSignalObject=off  FilterRTWStateStorageClass=Auto  ParallelPVariant=Passthrough  IdealPVariant=InternalParameters  IVariant=InternalParameters  DVariant=Disabled  IntegratorVariant=Continuous  SatVariant=Disabled  AWVariant=Passthrough  PCopyVariant=Disabled  TRVariant=Disabled  FdbkBlocksVariant=Forward  IdealPFdbkVariant=Disabled  SatFdbkVariant=Disabled  DerivativeFilterVariant=Disabled  NVariant=Disabled  NCopyVariant=Disabled_SignalSpec  FilterICVariant=Disabled  IntegratorICVariant=InternalICs  ExternalResetVariant=Disabled  TRSumVariant=Passthrough  SumFdbkVariant=Disabled  SumVariant=Sum_PI  TsampFilterVariant=InternalTs  TsampNgainVariant=Passthrough  TsampIntegralVariant=Disabled_SignalSpec  ExternalSaturationOutDataTypeStr=Inherit: Same as second input  DerivativeSourceVariant=Disabled  PreIntVariant=InternalPreInt
  Product : Product
  Relational Operator : RelationalOperator  Operator=<=  OutDataTypeStr=boolean  RndMeth=Simplest  InputSameDT=off
  Sum1 : Sum  Inputs=|++
  Switch : Switch  Criteria=u2 > Threshold  SaturateOnIntegerOverflow=off  InputSameDT=off
  Switch1 : Switch  Criteria=u2 > Threshold  SaturateOnIntegerOverflow=off  InputSameDT=off
  Switch2 : Switch  Criteria=u2 > Threshold  SaturateOnIntegerOverflow=off  InputSameDT=off
  ABS Torque OUT : Outport
  wires:
  Product/1 -> ABS Torque OUT/1  "Torq OUT"
  Switch/1 -> Sum1/2  "Ref Slip Ratio"
  Constant/1 -> Relational Operator/1
  Sum1/1 -> Switch1/1  "Slip Ratio Delta"
  Switch1/1 -> PID Controller/1
  PID Controller/1 -> Switch2/1
  Constant2/1 -> Switch/3
  Gain/1 -> Relational Operator/2
  Switch2/1 -> Product/2
  Constant4/1 -> Switch2/3
  Torque IN/1 -> Product/1  "Torque IN"
  Constant1/1 -> Switch/2, Switch/1
  Constant3/1 -> Switch1/3
  Relational Operator/1 -> Switch2/2, Switch1/2
  Slip_Ratio/1 -> Gain/1, Sum1/1  "Slip Ratio"

== system Rebuild/Main/Powertrain/Motors/Control Algorithms/ABS/ABS_FR ==
  Torque IN : Inport
  Slip_Ratio : Inport  Port=2
  Constant : Constant  Value=0.1
  Constant1 : Constant  Value=0.1
  Constant2 : Constant  Value=0.2
  Constant3 : Constant  Value=0
  Constant4 : Constant
  Gain : Gain  Gain=-1
  PID Controller : slpidlib/PID Controller  Controller=PI  Form=Ideal  TimeDomain=Continuous-time  UseExternalTs=off  SampleTime=-1  IntegratorMethod=Forward Euler  FilterMethod=Forward Euler  ControllerParametersSource=internal  P=100  I=10  UseKiTs=on  D=1  UseExternalDerivativeSource=off  N=100  UseFilter=on  TunerSelectOption=Transfer Function Based (PID Tuner App)  InitialConditionSource=internal  InitialConditionForIntegrator=0  InitialConditionForFilter=0  DifferentiatorICPrevScaledInput=0  ExternalReset=none  TrackingMode=off  Kt=1  LimitOutput=off  SatLimitsSource=internal  UpperSaturationLimit=inf  LowerSaturationLimit=-inf  LinearizeAsGain=on  AntiWindupMode=none  Kb=1  LimitIntegrator=off  UpperIntegratorSaturationLimit=inf  LowerIntegratorSaturationLimit=-inf  POutMin=[]  POutMax=[]  IOutMin=[]  IOutMax=[]  DOutMin=[]  DOutMax=[]  NOutMin=[]  NOutMax=[]  SumOutMin=[]  SumOutMax=[]  SaturationOutMin=[]  SaturationOutMax=[]  PParamMin=[]  PParamMax=[]  IParamMin=[]  IParamMax=[]  DParamMin=[]  DParamMax=[]  NParamMin=[]  NParamMax=[]  KbParamMin=[]  KbParamMax=[]  KtParamMin=[]  KtParamMax=[]  KbOutMin=[]  KbOutMax=[]  KtOutMin=[]  KtOutMax=[]  IntegratorOutMin=[]  IntegratorOutMax=[]  FilterOutMin=[]  FilterOutMax=[]  SumI1OutMin=[]  SumI1OutMax=[]  SumI2OutMin=[]  SumI2OutMax=[]  SumI3OutMin=[]  SumI3OutMax=[]  SumI4OutMin=[]  SumI4OutMax=[]  SumDOutMin=[]  SumDOutMax=[]  DifferentiatorOutMin=[]  DifferentiatorOutMax=[]  FilterDiffOutCoefMin=[]  FilterDiffOutCoefMax=[]  ReciprocalOutMin=[]  ReciprocalOutMax=[]  SumDenOutMin=[]  SumDenOutMax=[]  SumNumOutMin=[]  SumNumOutMax=[]  DivideOutMin=[]  DivideOutMax=[]  UdiffTsProdOutMin=[]  UdiffTsProdOutMax=[]  NTsProdOutMin=[]  NTsProdOutMax=[]  UintegralTsProdOutMin=[]  UintegralTsProdOutMax=[]  UngainTsProdOutMin=[]  UngainTsProdOutMax=[]  ClampingZeroOutDataTypeStr=Inherit: Inherit via back propagation  ClampingZeroOutMin=[]  ClampingZeroOutMax=[]  FilterDenConstantOutDataTypeStr=Inherit: Inherit via back propagation  FilterDenConstantOutMin=[]  FilterDenConstantOutMax=[]  PCopyOutDataTypeStr=Inherit: Inherit via back propagation  PCopyOutMin=[]  PCopyOutMax=[]  NCopyOutDataTypeStr=Inherit: Inherit via back propagation  NCopyOutMin=[]  NCopyOutMax=[]  IntegratorContinuousStateAttributes=''  IntegratorStateMustResolveToSignalObject=off  IntegratorRTWStateStorageClass=Auto  FilterContinuousStateAttributes=''  FilterStateMustResolveToSignalObject=off  FilterRTWStateStorageClass=Auto  ParallelPVariant=Passthrough  IdealPVariant=InternalParameters  IVariant=InternalParameters  DVariant=Disabled  IntegratorVariant=Continuous  SatVariant=Disabled  AWVariant=Passthrough  PCopyVariant=Disabled  TRVariant=Disabled  FdbkBlocksVariant=Forward  IdealPFdbkVariant=Disabled  SatFdbkVariant=Disabled  DerivativeFilterVariant=Disabled  NVariant=Disabled  NCopyVariant=Disabled_SignalSpec  FilterICVariant=Disabled  IntegratorICVariant=InternalICs  ExternalResetVariant=Disabled  TRSumVariant=Passthrough  SumFdbkVariant=Disabled  SumVariant=Sum_PI  TsampFilterVariant=InternalTs  TsampNgainVariant=Passthrough  TsampIntegralVariant=Disabled_SignalSpec  ExternalSaturationOutDataTypeStr=Inherit: Same as second input  DerivativeSourceVariant=Disabled  PreIntVariant=InternalPreInt
  Product : Product
  Relational Operator : RelationalOperator  Operator=<=  OutDataTypeStr=boolean  RndMeth=Simplest  InputSameDT=off
  Sum1 : Sum  Inputs=|++
  Switch : Switch  Criteria=u2 > Threshold  SaturateOnIntegerOverflow=off  InputSameDT=off
  Switch1 : Switch  Criteria=u2 > Threshold  SaturateOnIntegerOverflow=off  InputSameDT=off
  Switch2 : Switch  Criteria=u2 > Threshold  SaturateOnIntegerOverflow=off  InputSameDT=off
  ABS Torque OUT : Outport
  wires:
  Product/1 -> ABS Torque OUT/1  "Torq OUT"
  Switch/1 -> Sum1/2  "Ref Slip Ratio"
  Constant/1 -> Relational Operator/1
  Sum1/1 -> Switch1/1  "Slip Ratio Delta"
  Switch1/1 -> PID Controller/1
  PID Controller/1 -> Switch2/1
  Constant2/1 -> Switch/3
  Gain/1 -> Relational Operator/2
  Switch2/1 -> Product/2
  Constant4/1 -> Switch2/3
  Torque IN/1 -> Product/1  "Torque IN"
  Constant1/1 -> Switch/2, Switch/1
  Constant3/1 -> Switch1/3
  Relational Operator/1 -> Switch2/2, Switch1/2
  Slip_Ratio/1 -> Gain/1, Sum1/1  "Slip Ratio"

== system Rebuild/Main/Powertrain/Motors/Control Algorithms/ABS/ABS_RL ==
  Torque IN : Inport
  Slip_Ratio : Inport  Port=2
  Constant : Constant  Value=0.1
  Constant1 : Constant  Value=0.1
  Constant2 : Constant  Value=0.2
  Constant3 : Constant  Value=0
  Constant4 : Constant
  Gain : Gain  Gain=-1
  PID Controller : slpidlib/PID Controller  Controller=PI  Form=Ideal  TimeDomain=Continuous-time  UseExternalTs=off  SampleTime=-1  IntegratorMethod=Forward Euler  FilterMethod=Forward Euler  ControllerParametersSource=internal  P=100  I=10  UseKiTs=on  D=1  UseExternalDerivativeSource=off  N=100  UseFilter=on  TunerSelectOption=Transfer Function Based (PID Tuner App)  InitialConditionSource=internal  InitialConditionForIntegrator=0  InitialConditionForFilter=0  DifferentiatorICPrevScaledInput=0  ExternalReset=none  TrackingMode=off  Kt=1  LimitOutput=off  SatLimitsSource=internal  UpperSaturationLimit=inf  LowerSaturationLimit=-inf  LinearizeAsGain=on  AntiWindupMode=none  Kb=1  LimitIntegrator=off  UpperIntegratorSaturationLimit=inf  LowerIntegratorSaturationLimit=-inf  POutMin=[]  POutMax=[]  IOutMin=[]  IOutMax=[]  DOutMin=[]  DOutMax=[]  NOutMin=[]  NOutMax=[]  SumOutMin=[]  SumOutMax=[]  SaturationOutMin=[]  SaturationOutMax=[]  PParamMin=[]  PParamMax=[]  IParamMin=[]  IParamMax=[]  DParamMin=[]  DParamMax=[]  NParamMin=[]  NParamMax=[]  KbParamMin=[]  KbParamMax=[]  KtParamMin=[]  KtParamMax=[]  KbOutMin=[]  KbOutMax=[]  KtOutMin=[]  KtOutMax=[]  IntegratorOutMin=[]  IntegratorOutMax=[]  FilterOutMin=[]  FilterOutMax=[]  SumI1OutMin=[]  SumI1OutMax=[]  SumI2OutMin=[]  SumI2OutMax=[]  SumI3OutMin=[]  SumI3OutMax=[]  SumI4OutMin=[]  SumI4OutMax=[]  SumDOutMin=[]  SumDOutMax=[]  DifferentiatorOutMin=[]  DifferentiatorOutMax=[]  FilterDiffOutCoefMin=[]  FilterDiffOutCoefMax=[]  ReciprocalOutMin=[]  ReciprocalOutMax=[]  SumDenOutMin=[]  SumDenOutMax=[]  SumNumOutMin=[]  SumNumOutMax=[]  DivideOutMin=[]  DivideOutMax=[]  UdiffTsProdOutMin=[]  UdiffTsProdOutMax=[]  NTsProdOutMin=[]  NTsProdOutMax=[]  UintegralTsProdOutMin=[]  UintegralTsProdOutMax=[]  UngainTsProdOutMin=[]  UngainTsProdOutMax=[]  ClampingZeroOutDataTypeStr=Inherit: Inherit via back propagation  ClampingZeroOutMin=[]  ClampingZeroOutMax=[]  FilterDenConstantOutDataTypeStr=Inherit: Inherit via back propagation  FilterDenConstantOutMin=[]  FilterDenConstantOutMax=[]  PCopyOutDataTypeStr=Inherit: Inherit via back propagation  PCopyOutMin=[]  PCopyOutMax=[]  NCopyOutDataTypeStr=Inherit: Inherit via back propagation  NCopyOutMin=[]  NCopyOutMax=[]  IntegratorContinuousStateAttributes=''  IntegratorStateMustResolveToSignalObject=off  IntegratorRTWStateStorageClass=Auto  FilterContinuousStateAttributes=''  FilterStateMustResolveToSignalObject=off  FilterRTWStateStorageClass=Auto  ParallelPVariant=Passthrough  IdealPVariant=InternalParameters  IVariant=InternalParameters  DVariant=Disabled  IntegratorVariant=Continuous  SatVariant=Disabled  AWVariant=Passthrough  PCopyVariant=Disabled  TRVariant=Disabled  FdbkBlocksVariant=Forward  IdealPFdbkVariant=Disabled  SatFdbkVariant=Disabled  DerivativeFilterVariant=Disabled  NVariant=Disabled  NCopyVariant=Disabled_SignalSpec  FilterICVariant=Disabled  IntegratorICVariant=InternalICs  ExternalResetVariant=Disabled  TRSumVariant=Passthrough  SumFdbkVariant=Disabled  SumVariant=Sum_PI  TsampFilterVariant=InternalTs  TsampNgainVariant=Passthrough  TsampIntegralVariant=Disabled_SignalSpec  ExternalSaturationOutDataTypeStr=Inherit: Same as second input  DerivativeSourceVariant=Disabled  PreIntVariant=InternalPreInt
  Product : Product
  Relational Operator : RelationalOperator  Operator=<=  OutDataTypeStr=boolean  RndMeth=Simplest  InputSameDT=off
  Sum1 : Sum  Inputs=|++
  Switch : Switch  Criteria=u2 > Threshold  SaturateOnIntegerOverflow=off  InputSameDT=off
  Switch1 : Switch  Criteria=u2 > Threshold  SaturateOnIntegerOverflow=off  InputSameDT=off
  Switch2 : Switch  Criteria=u2 > Threshold  SaturateOnIntegerOverflow=off  InputSameDT=off
  ABS Torque OUT : Outport
  wires:
  Product/1 -> ABS Torque OUT/1  "Torq OUT"
  Switch/1 -> Sum1/2  "Ref Slip Ratio"
  Constant/1 -> Relational Operator/1
  Sum1/1 -> Switch1/1  "Slip Ratio Delta"
  Switch1/1 -> PID Controller/1
  PID Controller/1 -> Switch2/1
  Constant2/1 -> Switch/3
  Gain/1 -> Relational Operator/2
  Switch2/1 -> Product/2
  Constant4/1 -> Switch2/3
  Torque IN/1 -> Product/1  "Torque IN"
  Constant1/1 -> Switch/2, Switch/1
  Constant3/1 -> Switch1/3
  Relational Operator/1 -> Switch2/2, Switch1/2
  Slip_Ratio/1 -> Gain/1, Sum1/1  "Slip Ratio"
